simulink model "mcb_pmsm_foc_sensorless_dsPIC33EP256MC506"  (R2021b)
settings: Solver=FixedStepDiscrete  StartTime=0.0  StopTime=10  FixedStep=Ts  RelTol=1e-3  EnableMultiTasking=on
InitFcn:
  | mcb_pmsm_foc_sensorless_dsPIC33_data;
values from neighbouring files (symbols this model uses):
  dataType = fixdt(1,16,14)    [mcb_pmsm_foc_sensorless_dsPIC33_data.m]
  dataType2 = fixdt(1,16,12)    [mcb_pmsm_foc_sensorless_dsPIC33_data.m]
  PI_params = mcb.internal.SetControllerParameters(pmsm,inverter,PU_System,T_pwm,Ts,Ts_speed)    [mcb_pmsm_foc_sensorless_dsPIC33_data.m]
  PU_System = mcb_SetPUSystem(pmsm,inverter)    [mcb_pmsm_foc_sensorless_dsPIC33_data.m]
  PWM_frequency = 20e3    (= 20000)    [mcb_pmsm_foc_sensorless_dsPIC33_data.m]
  Speed_openLoop_PU = 0.1    [mcb_pmsm_foc_sensorless_dsPIC33_data.m]
  Ts = T_pwm    (= 5e-05)    [mcb_pmsm_foc_sensorless_dsPIC33_data.m]
  Ts_speed = 30*Ts    (= 0.0015)    [mcb_pmsm_foc_sensorless_dsPIC33_data.m]
undefined symbols (not defined in the file or in its folder): A4, C5, D8, F1, inverter, P20, P53, P97, Pin, pmsm, PWMmax
libraries: MCHP_Blockset x16, mcbcontrolslib x13, simulink x9, mcbpositiondecoderlib x2, mcbplantlib x1, autolibpmsmexterior x1
(part 3 of 3)

== system mcb_pmsm_foc_sensorless_dsPIC33EP256MC506/Current Control/To Matlab Host /Serial Send/SCI_Tx/End ==
  Data : Inport
  Action Port : ActionPort  ActionPortLabel=elseif(u1 == 599)
  Mux : Mux  Inputs=2
  Start : Constant  Value=hex2dec('45')  OutDataTypeStr=uint8
  UART Tx : MCHP_Blockset/BUS UART/UART Tx  UART_REF=2  ORDERING=None  AllOrNothing=off  SampleTime=-1  MCHP_MASTERLINK=mcb_pmsm_foc_sensorless_dsPIC33EP256MC506/Hardware Init/Microchip Master  NSend_Input=off  UART_String=off  NSend_Output=off
      settings: SourceProductName=MPLAB Device Blocks for Simulink
  wires:
  Mux/1 -> UART Tx/1
  Data/1 -> Mux/1
  Start/1 -> Mux/2

== system mcb_pmsm_foc_sensorless_dsPIC33EP256MC506/Current Control/To Matlab Host /Serial Send/SCI_Tx/Start ==
  Data : Inport
  Action Port : ActionPort  ActionPortLabel=if(u1 == 0)
  End : Constant  Value=hex2dec('53')  OutDataTypeStr=uint8
  Mux : Mux  Inputs=2
  UART Tx : MCHP_Blockset/BUS UART/UART Tx  UART_REF=2  ORDERING=None  AllOrNothing=off  SampleTime=-1  MCHP_MASTERLINK=mcb_pmsm_foc_sensorless_dsPIC33EP256MC506/Hardware Init/Microchip Master  NSend_Input=off  UART_String=off  NSend_Output=off
      settings: SourceProductName=MPLAB Device Blocks for Simulink
  wires:
  Mux/1 -> UART Tx/1
  Data/1 -> Mux/2
  End/1 -> Mux/1

== system mcb_pmsm_foc_sensorless_dsPIC33EP256MC506/Current Control/Input Scaling/Sensorless/Flux Observer2/psiAlpha/Hhp ==
  Input : Inport
  A2Delay1 : Delay  DelayLength=1  InitialCondition=0
  B2Delay1 : Delay  DelayLength=1  InitialCondition=0
  CastStates1 : DataTypeConversion  OutDataTypeStr=fixdt(1,16,13)  SaturateOnIntegerOverflow=on  RndMeth=Zero
  ConvertIn : DataTypeConversion  OutDataTypeStr=fixdt(1,16,13)  RndMeth=Nearest  SaturateOnIntegerOverflow=on
  ConvertScale1 : DataTypeConversion  OutDataTypeStr=fixdt(1,16,13)  SaturateOnIntegerOverflow=on  RndMeth=Zero
  SumA21 : Sum  Inputs=|+-  AccumDataTypeStr=fixdt(1,32,25)  OutDataTypeStr=fixdt(1,32,25)  RndMeth=Zero  SaturateOnIntegerOverflow=on
  SumB21 : Sum  Inputs=|++  AccumDataTypeStr=fixdt(1,32,26)  OutDataTypeStr=fixdt(1,32,26)  RndMeth=Zero  SaturateOnIntegerOverflow=on
  a(2)(1) : Gain  Gain=-0.995470563986853518  ParamDataTypeStr=fixdt(1,16,14)  OutDataTypeStr=fixdt(1,32,27)  RndMeth=Zero  SaturateOnIntegerOverflow=on
  b(1)(1) : Gain  Gain=0.99773528199352135  ParamDataTypeStr=fixdt(1,16,15)  OutDataTypeStr=fixdt(1,32,28)  RndMeth=Zero  SaturateOnIntegerOverflow=on
  b(2)(1) : Gain  Gain=-0.99773528199352135  ParamDataTypeStr=fixdt(1,16,15)  OutDataTypeStr=fixdt(1,32,28)  RndMeth=Zero  SaturateOnIntegerOverflow=on
  s(2) : Gain  Gain=0.999999999999905187  ParamDataTypeStr=fixdt(1,16,15)  OutDataTypeStr=fixdt(1,16,9)  RndMeth=Zero  SaturateOnIntegerOverflow=on
  Output : Outport
  wires:
  Input/1 -> ConvertIn/1
  ConvertScale1/1 -> b(1)(1)/1, B2Delay1/1
  b(1)(1)/1 -> SumB21/1
  SumB21/1 -> SumA21/1
  SumA21/1 -> CastStates1/1
  CastStates1/1 -> s(2)/1, A2Delay1/1
  B2Delay1/1 -> b(2)(1)/1
  b(2)(1)/1 -> SumB21/2
  a(2)(1)/1 -> SumA21/2
  A2Delay1/1 -> a(2)(1)/1
  s(2)/1 -> Output/1
  ConvertIn/1 -> ConvertScale1/1

== system mcb_pmsm_foc_sensorless_dsPIC33EP256MC506/Current Control/Input Scaling/Sensorless/Flux Observer2/psiAlpha/Scaling ==
  "Valpha " : Inport
  Ialpha : Inport  Port=2
  ScalingL : Gain  Gain=StatorDAxisInductance*PerUnitCurrent/PerUnitVoltage  OutMin=-StatorDAxisInductance*PerUnitCurrent/PerUnitVoltage  OutMax=StatorDAxisInductance*PerUnitCurrent/PerUnitVoltage  OutDataTypeStr=fixdt(1,16)  RndMeth=Zero
  ScalingR : Gain  Gain=StatorResistance*PerUnitCurrent/PerUnitVoltage  OutMin=-StatorResistance*PerUnitCurrent/PerUnitVoltage  OutMax=StatorResistance*PerUnitCurrent/PerUnitVoltage  OutDataTypeStr=fixdt(1,16)  RndMeth=Zero
  ValphaScaled : Outport
  IalphaScaled*R : Outport  Port=2
  IalphaScaled*L : Outport  Port=3
  wires:
  Ialpha/1 -> ScalingR/1, ScalingL/1
  ScalingL/1 -> IalphaScaled*L/1
  "Valpha "/1 -> ValphaScaled/1
  ScalingR/1 -> IalphaScaled*R/1

== system mcb_pmsm_foc_sensorless_dsPIC33EP256MC506/Current Control/Input Scaling/Sensorless/Flux Observer2/psiBeta/Hhp ==
  Input : Inport
  A2Delay1 : Delay  DelayLength=1  InitialCondition=0
  B2Delay1 : Delay  DelayLength=1  InitialCondition=0
  CastStates1 : DataTypeConversion  OutDataTypeStr=fixdt(1,16,13)  SaturateOnIntegerOverflow=on  RndMeth=Zero
  ConvertIn : DataTypeConversion  OutDataTypeStr=fixdt(1,16,13)  RndMeth=Nearest  SaturateOnIntegerOverflow=on
  ConvertScale1 : DataTypeConversion  OutDataTypeStr=fixdt(1,16,13)  SaturateOnIntegerOverflow=on  RndMeth=Zero
  SumA21 : Sum  Inputs=|+-  AccumDataTypeStr=fixdt(1,32,25)  OutDataTypeStr=fixdt(1,32,25)  RndMeth=Zero  SaturateOnIntegerOverflow=on
  SumB21 : Sum  Inputs=|++  AccumDataTypeStr=fixdt(1,32,26)  OutDataTypeStr=fixdt(1,32,26)  RndMeth=Zero  SaturateOnIntegerOverflow=on
  a(2)(1) : Gain  Gain=-0.995470563986853518  ParamDataTypeStr=fixdt(1,16,14)  OutDataTypeStr=fixdt(1,32,27)  RndMeth=Zero  SaturateOnIntegerOverflow=on
  b(1)(1) : Gain  Gain=0.99773528199352135  ParamDataTypeStr=fixdt(1,16,15)  OutDataTypeStr=fixdt(1,32,28)  RndMeth=Zero  SaturateOnIntegerOverflow=on
  b(2)(1) : Gain  Gain=-0.99773528199352135  ParamDataTypeStr=fixdt(1,16,15)  OutDataTypeStr=fixdt(1,32,28)  RndMeth=Zero  SaturateOnIntegerOverflow=on
  s(2) : Gain  Gain=0.999999999999905187  ParamDataTypeStr=fixdt(1,16,15)  OutDataTypeStr=fixdt(1,16,9)  RndMeth=Zero  SaturateOnIntegerOverflow=on
  Output : Outport
  wires:
  Input/1 -> ConvertIn/1
  ConvertScale1/1 -> b(1)(1)/1, B2Delay1/1
  b(1)(1)/1 -> SumB21/1
  SumB21/1 -> SumA21/1
  SumA21/1 -> CastStates1/1
  CastStates1/1 -> s(2)/1, A2Delay1/1
  B2Delay1/1 -> b(2)(1)/1
  b(2)(1)/1 -> SumB21/2
  a(2)(1)/1 -> SumA21/2
  A2Delay1/1 -> a(2)(1)/1
  s(2)/1 -> Output/1
  ConvertIn/1 -> ConvertScale1/1

== system mcb_pmsm_foc_sensorless_dsPIC33EP256MC506/Current Control/Input Scaling/Sensorless/Flux Observer2/psiBeta/Scaling ==
  Vbeta : Inport
  Ibeta : Inport  Port=2
  ScalingL : Gain  Gain=StatorDAxisInductance*PerUnitCurrent/PerUnitVoltage  OutMin=-StatorDAxisInductance*PerUnitCurrent/PerUnitVoltage  OutMax=StatorDAxisInductance*PerUnitCurrent/PerUnitVoltage  OutDataTypeStr=fixdt(1,16)  RndMeth=Zero
  ScalingR : Gain  Gain=StatorResistance*PerUnitCurrent/PerUnitVoltage  OutMin=-StatorResistance*PerUnitCurrent/PerUnitVoltage  OutMax=StatorResistance*PerUnitCurrent/PerUnitVoltage  OutDataTypeStr=fixdt(1,16)  RndMeth=Zero
  VbetaScaled : Outport
  IbetaScaled*R : Outport  Port=2
  IbetaScaled*L : Outport  Port=3
  wires:
  Ibeta/1 -> ScalingR/1, ScalingL/1
  ScalingL/1 -> IbetaScaled*L/1
  Vbeta/1 -> VbetaScaled/1
  ScalingR/1 -> IbetaScaled*R/1

== stateflow chart mcb_pmsm_foc_sensorless_dsPIC33EP256MC506/Current Control/Closed Loop Control/Open_Loop_Control/OpentoClosed/Chart ==
  state Init
    during: Mode = 0;
    SpeedCtrl = 0;
  state Align
    during: Mode = 0;
    SpeedCtrl = 0;
  state ClosedLoopFilter
    during: Mode = 2;
    SpeedCtrl = 1;
  state ClosedLoop
    during: Mode = 2;
    SpeedCtrl = 0;
  state OpenLoop
    during: Mode = 1;
    SpeedCtrl = 0;
  (default) -> Init
  ClosedLoopFilter -> Init : [En == 0]
  ClosedLoop -> Init [order 1] : [En == 0]
  Init -> Align : [En == 1]
  Align -> Init [order 1] : [En == 0]
  OpenLoop -> Init [order 2] : [En == 0]
  Align -> OpenLoop [order 2] : after(0.5,sec)
  ClosedLoop -> ClosedLoopFilter [order 2] : after(0.1,sec)
  OpenLoop -> ClosedLoop [order 1] : after(0.5,sec)[SpeedFb > Limit]
  data: Limit input fixdt(1,16,14); SpeedFb input fixdt(1,16,14); Mode output uint16; En input boolean; SpeedCtrl output uint16
